simulink model "pathPlanningBicycleSimulinkModel"  (R2021a)
settings: Solver=VariableStepAuto  StartTime=0.0  StopTime=10000  RelTol=1e-3
model workspace (MAT data in the model file):
  Sig = Simulink.Signal
  Sig.DataType = 'auto'
  Sig.Dimensions = -1
  Sig.DimensionsMode = 'auto'
  Sig.Complexity = 'auto'
  Sig.SampleTime = -1
  Sig.SamplingMode = 'auto'
undefined symbols (not defined in the file or in its folder): chosenMap, goalLoc, startLoc, startOrient
libraries: robotmobilelib x1, robotalgslib x1
settings Model: OrderedModelArguments=off  Creator=The MathWorks, Inc.  LastModifiedBy=User
settings SolverCC: AlgebraicLoopSolver=TrustRegion
settings DebuggingCC: SymbolicDimsDataTypeCodeGenerationDiagnostic=none  SFMachineParentedDataDiag=warning

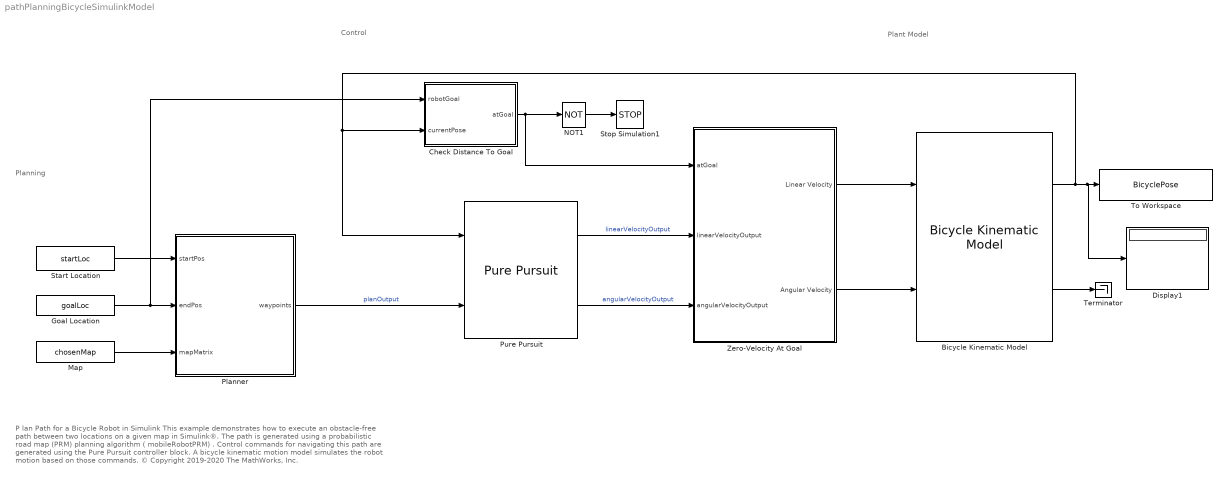
== system pathPlanningBicycleSimulinkModel ==
  note: Control
  note: Plant Model
  note: Planning
  note: P lan Path for a Bicycle Robot in Simulink
      | This example demonstrates how to execute an obstacle-free path between two locations on a given map in Simulink®. The path is generated using a probabilistic road map (PRM) planning algorithm ( mobileRobotPRM) . Control commands for navigating this path are generated using the Pure Pursuit controller block. A bicycle kinematic motion model simulates the robot motion based on those commands.
      |
      | © Copyright 2019-2020 The MathWorks, Inc.
  Bicycle Kinematic Model : robotmobilelib/Bicycle Kinematic Model  VehicleInputs=Vehicle Speed & Heading Angular Velocity  WheelBase=1  VehicleSpeedRange=[-inf, inf]  MaxSteeringAngle=pi/2  InitialState=[startLoc startOrient]  SimulateUsing=Interpreted execution
      settings: SourceProductBaseCode=RO
  Check Distance To Goal : Subsystem
  Display1 : Display
  Goal Location : Constant  Value=goalLoc
  Map : Constant  Value=chosenMap
  NOT1 : Logic  Operator=NOT  IconShape=distinctive  AllPortsSameDT=off  OutDataTypeStr=boolean
  Planner : MATLAB Function  TreatAsAtomicUnit=on
  Pure Pursuit : robotalgslib/Pure Pursuit  DesiredLinearVelocity=0.1  MaxAngularVelocity=1.0  LookaheadDistance=0.5  TargetDirPort=off  SimulateUsing=Code generation
  Start Location : Constant  Value=startLoc
  Stop Simulation1 : Stop
  Terminator : Terminator
  To Workspace : ToWorkspace  VariableName=BicyclePose  SampleTime=-1
  Zero-Velocity At Goal : Subsystem
  wires:
  Planner/1(waypoints) -> Pure Pursuit/2  "planOutput"
  Start Location/1 -> Planner/1(startPos)
  Goal Location/1 -> Check Distance To Goal/1(robotGoal), Planner/2(endPos)
  Map/1 -> Planner/3(mapMatrix)
  Check Distance To Goal/1(atGoal) -> Zero-Velocity At Goal/1(atGoal), NOT1/1
  Bicycle Kinematic Model/1 -> Pure Pursuit/1, Check Distance To Goal/2(currentPose), Display1/1, To Workspace/1
  Zero-Velocity At Goal/2(Angular Velocity) -> Bicycle Kinematic Model/2
  NOT1/1 -> Stop Simulation1/1
  Pure Pursuit/1 -> Zero-Velocity At Goal/2(linearVelocityOutput)  "linearVelocityOutput"
  Bicycle Kinematic Model/2 -> Terminator/1
  Pure Pursuit/2 -> Zero-Velocity At Goal/3(angularVelocityOutput)  "angularVelocityOutput"
  Zero-Velocity At Goal/1(Linear Velocity) -> Bicycle Kinematic Model/1

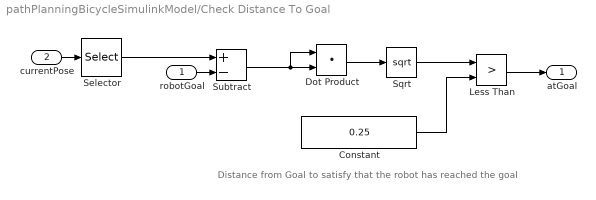
== system pathPlanningBicycleSimulinkModel/Check Distance To Goal ==
  note: Distance from Goal to satisfy that the robot has reached the goal
  robotGoal : Inport
  currentPose : Inport  Port=2
  Constant : Constant  Value=0.25
  Dot Product : DotProduct  InputSameDT=on  OutDataTypeStr=Inherit: Inherit via internal rule
  Less Than : RelationalOperator  Operator=>  OutDataTypeStr=boolean  RndMeth=Simplest
  Selector : Selector  InputPortWidth=3  IndexOptions=Index vector (dialog)  Indices=[1 2]  OutputSizes=1
  Sqrt : Sqrt  SaturateOnIntegerOverflow=on
  Subtract : Sum  Inputs=+-
  atGoal : Outport
  wires:
  robotGoal/1 -> Subtract/2
  Dot Product/1 -> Sqrt/1
  Constant/1 -> Less Than/2
  currentPose/1 -> Selector/1
  Less Than/1 -> atGoal/1
  Sqrt/1 -> Less Than/1
  Subtract/1 -> Dot Product/1, Dot Product/2
  Selector/1 -> Subtract/1

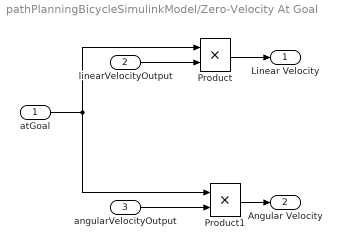
== system pathPlanningBicycleSimulinkModel/Zero-Velocity At Goal ==
  atGoal : Inport
  linearVelocityOutput : Inport  Port=2
  angularVelocityOutput : Inport  Port=3
  Product : Product
  Product1 : Product
  Linear Velocity : Outport  OutDataTypeStr=double
  Angular Velocity : Outport  Port=2  OutDataTypeStr=double
  wires:
  atGoal/1 -> Product1/1, Product/1
  angularVelocityOutput/1 -> Product1/2
  linearVelocityOutput/1 -> Product/2
  Product/1 -> Linear Velocity/1
  Product1/1 -> Angular Velocity/1

== matlab function pathPlanningBicycleSimulinkModel/Planner ==
  settings: updateMethod=DISCRETE
  data: startPos input size=[1 2]; endPos input size=[1 2]; waypoints output size=[100 2]; mapMatrix input
function waypoints = planning(startPos, endPos, mapMatrix)
% persistent creates a variable used only in the function, but that keeps
% its value in the next call of the function
persistent waypointsInternal
persistent prevStartPos
persistent prevEndPos

% Set constant parameters
maxNumNodes = 100;

% Initialize persistent variables that are used downstream
if isempty(prevStartPos)
    prevStartPos = startPos;
end

if isempty(prevEndPos)
    prevEndPos = endPos;
end

isNewPath = (~isequal(prevStartPos, startPos) || ~isequal(prevEndPos, endPos));

if isempty(waypointsInternal) || isNewPath
    % Two conditions in which waypoints must be set: they are not yet
    % initialized, or they are initialized, but the current start and end
    % do not match those used to generate the previous set of waypoints
    [waypointsInternal] = planPath(mapMatrix, maxNumNodes, startPos, endPos);
end

% Update the outputs
waypoints = waypointsInternal;

% Update the persistent variables that indicate previous state
prevStartPos = startPos;
prevEndPos = endPos;

%% Helper Function

function wayPoints = planPath(mapMatrix, maxNodes, startPos, endPos)
    
    % Create a probabilistic roadmap
    map = binaryOccupancyMap(mapMatrix);
    prm = mobileRobotPRM(map, maxNodes);
    
    % Find a path between two points
    xy = findpath(prm, startPos, endPos);
    wayPoints = repmat(endPos, maxNodes, 1);
    
    % Number of nodes that are actually used
    numNodes = length(xy);
    wayPoints(1:numNodes,:) = xy;    

end

end
